simulink model "ISReferenceApplication"  (R2019b)
settings: Solver=VariableStepAuto  StartTime=0.0  StopTime=10.0  RelTol=1e-3
undefined symbols (not defined in the file or in its folder): C_Brake, C_Final, C_Front, C_Middle, C_out_Brake, C_out_Final, C_out_Front, C_out_Middle, Co, Cso, D_out_Brake, D_out_Final, D_out_Front, D_out_Middle, Downshift_Speeds, F, F_Brake, F_Final, F_Front, F_Middle, Fs, G_Brake, G_Final, G_Front, G_Middle, G_sys_Brake, G_sys_Final, G_sys_Front, G_sys_Middle, Gd, Gd_Brake, Gd_Final, Gsd, h, H_Brake, H_Final, H_Front, H_Middle, H_sys_Brake, H_sys_Final, H_sys_Front, H_sys_Middle, Hd, Hd_Brake, Hd_Final, Hsd, JE, JE_Brake, JE_Final, JE_Front, JE_Middle, JEs, JF_part, JF_part_Brake, JF_part_Final, JF_parts, Ld, Ld_Brake, Ld_Final, Ld_Front ... (+21)
libraries: simulink x5, autolibutils x3, sim3dlib x2, vehdynlibviscommon x1
(part 4 of 4)

== matlab function ISReferenceApplication/Final Observer2/Subsystem/Pose updete k/Update ==
  settings: updateMethod=DISCRETE  sampleTime=Ts
  data: Rs_V_now input; Rs_Y_now input; XYline input; XYplot input; XYplot_sim input; Last_XYplot_sim input; Velocity_sim input; Last_Velocity_sim input; Heading_sim input; Last_Heading_sim input; Tsim input; Last_Heading_end input; Velocity_updated output; Heading_updated output [1..5]; Heading_end output
function [Velocity_updated, Heading_updated, Heading_end] = Y_update(Rs_V_now, Rs_Y_now, ...
        XYline, XYplot, XYplot_sim, Last_XYplot_sim, Velocity_sim, Last_Velocity_sim, Heading_sim, Last_Heading_sim, ... 
    Tsim, Last_Heading_end)
    disp(sprintf('Simulation time : %2.1f sec',Tsim)) 
    Np = 5; Ts = 0.1;
    Heading_updated = zeros(Np,1); Velocity_updated = zeros(Np,1);Heading_end = 0;
    coder.extrinsic('intersections');
    coder.extrinsic('P2YV');
%     coder.varsize('Velocity_updated_tmp',[5 1]);
%     coder.varsize('Heading_updated_tmp',[5 1]);
     if Tsim == 0 
        plot(XYline(:,2),XYline(:,1),'black');
    end
   

%%Create half-circle    

    N = 30;
    theta = zeros(Np-1,N+1); Veh_circle = zeros(N+1,(Np-1)*2); 
    xp = zeros(1,N+1); yp = zeros(1,N+1); X = [];  Y = []; X_tmp = 0; Y_tmp = 0;
    lookahead = zeros(Np-1,1);
    
    XYplot_sim_tmp = XYplot_sim;    

%     if Velocity_sim > 0.5
        Velocity_ahead = [Velocity_sim; Rs_V_now(2:Np-1,:)];
%     else
%         Velocity_ahead = Rs_V_now;
%     end

    lookahead = Velocity_ahead*Ts;
    Headngahead = [Heading_sim; Rs_Y_now(2:Np-1,:)];
%     lookahead = [1; 1.5; 2; 2.5; 3];
        
    for j = 1:Np-1        
        theta = Headngahead(j,:)-pi/4 : pi/2/N : Headngahead(j,:)+pi/4;
        xp = lookahead(j,:)*cos(theta) + XYplot_sim_tmp(1,:)*ones(1,length(theta));
        yp = lookahead(j,:)*sin(theta) + XYplot_sim_tmp(2,:)*ones(1,length(theta));
        Veh_circle(:,2*j-1:2*j) = [xp' yp'];
       
    %Find the intersection    
         
        [X_tmp, Y_tmp] = intersections(XYplot(:,1), XYplot(:,2), Veh_circle(:,2*j-1), Veh_circle(:,2*j),0); 
        
        if X_tmp == 0 && Y_tmp == 0
%             X = X_tmp(1:j-1,:);
%             Y = Y_tmp(1:j-1,:);
            break;
        end

        X = [X; X_tmp];
        Y = [Y; Y_tmp];   
        XYplot_sim_tmp = [X_tmp; Y_tmp];
        
    end 
    
%%Obtain predict Velocity and Heading angle
   
  
    
    X = [Last_XYplot_sim(1,:); XYplot_sim(1,:); X];
    Y = [Last_XYplot_sim(2,:); XYplot_sim(2,:); Y];
    Vx0 = Last_Velocity_sim*cos(Last_Heading_sim);
    Vy0 = Last_Velocity_sim*sin(Last_Heading_sim);
    Yaw0 = Last_Heading_sim;
     
    T_sample = []; 
    for j = 1:length(X)
        T_sample = [T_sample; Tsim+(j-1)*Ts];
    end
    
   [Velocity_updated, Heading_updated] = P2YV(0, T_sample , X , Y , Vx0 , Vy0 , Yaw0, Np, Last_Heading_end );
   Heading_end = Heading_updated(end,:);

%     Heading_tmp_end = atan2(XYplot(end,2)-XYplot_sim(2,:), XYplot(end,1)-XYplot_sim(1,:));
% 
%     if  ((Heading_tmp_end - Heading_tmp_end_delay) < -5/3*pi) % Angle compensation
%         Heading_flag_end = Heading_flag_end + 1;
%     elseif ((Heading_tmp_end - Heading_tmp_end_delay) > 5/3*pi)
%         Heading_flag_end = Heading_flag_end - 1;
%     end
%     
%     if flag == 1
%         Heading_updated(1:end) = Heading_tmp_end + Heading_flag_end*2*pi;
%     end
%     if Tsim == 1.5
%         figure();
%         plot(XYplot(:,2),XYplot(:,1),'black-');
%         hold on;
%         plot(XYplot_sim(2,:),XYplot_sim(1,:),'b o');
%         plot(Veh_circle(:,2), Veh_circle(:,1),'b-');
%         plot(Veh_circle(:,4), Veh_circle(:,3),'b-');
%         plot(Veh_circle(:,6), Veh_circle(:,5),'b-');
%         plot(Veh_circle(:,8), Veh_circle(:,7),'b-');
%         plot(Veh_circle(:,10), Veh_circle(:,9),'b-');
%         plot(Y, X,'r x');
%     end

end

== matlab function ISReferenceApplication/Final Observer2/Subsystem/VH2P/YV2P ==
  data: Velocity input; Yaw input; LastVelocity input; LastYaw input; Tsim input; LastTsim input; Lastpostion input; Position output
function Position  = YV2P(Velocity, Yaw,  LastVelocity, LastYaw, Tsim, LastTsim, Lastpostion)
if Tsim >= 0.1
    Position = zeros(2,1);
    X0 = Lastpostion(1,:); Y0 = Lastpostion(2,:);
    Vx = [LastVelocity*cos(LastYaw); Velocity*cos(Yaw)];
    Vy = [LastVelocity*sin(LastYaw); Velocity*sin(Yaw)];
    Yaw_sim = [LastYaw; Yaw];
    T_sample =[LastTsim; Tsim];
    [ X_tmp, Y_tmp] = YV2P( T_sample, X0, Y0, Vx, Vy, Yaw_sim, zeros(2,1) );
    Position = [X_tmp(end,:); Y_tmp(end,:)];
else
    Position = [0; 0];
end

end

== matlab function ISReferenceApplication/Final Observer2/Subsystem/YV_update_Np/MATLAB Function2 ==
  data: XY_ref input; Velocity_updated output; XY_sim input; LastXY_sim input; Velocity_sim input; LastVelocity_sim input; Yaw_sim input; LastYaw_sim input; Tsim input; Heading_updated output
function [Velocity_updated, Heading_updated] = VY_update(XY_ref, XY_sim, LastXY_sim, Velocity_sim, LastVelocity_sim, Yaw_sim, LastYaw_sim, Tsim)
    disp(sprintf('Simulation time : %2.1f sec',Tsim)) 
 Ts = 0.1;
% Np = 6;
 Np = 6;

 Heading_updated = zeros(Np,1); Velocity_updated = zeros(Np,1);
coder.extrinsic('P2YV');
% T_sample = [Tsim-0.01; Tsim; Tsim+0.01];
% X = [LastXY_sim(1); XY_sim(1); XY_ref(1,:)];
% Y = [LastXY_sim(2); XY_sim(2); XY_ref(2,:)];

% T_sample = [Tsim-0.01; Tsim; Tsim+0.01; Tsim+0.02];
% X = [LastXY_sim(1); XY_sim(1); XY_ref(1,:); XY_ref(3,:)];
% Y = [LastXY_sim(2); XY_sim(2); XY_ref(2,:); XY_ref(4,:)];

T_sample = []; 
for j = 1:Np+1
    T_sample = [T_sample; Tsim+(j-1)*Ts];
end
X = [];
for i = 1:Np
    X = [X; XY_ref(2*i-1,:)];
end
Y = [];
for i = 1:Np
    Y = [Y; XY_ref(2*i,:)];
end

X = [XY_sim(1,:); X];
Y = [XY_sim(2,:); Y];   
Vx0 = Velocity_sim*cos(Yaw_sim);
Vy0 = Velocity_sim*sin(Yaw_sim);
Yaw0 = Yaw_sim;

[Velocity_updated, Heading_updated] = P2YV(0,0, T_sample , X , Y , Vx0 , Vy0 , Yaw0, Np, 0, 0 );

end

== matlab function ISReferenceApplication/Final Observer2/Subsystem/VH2P/MATLAB Function1 ==
  data: select_model input; tri output
function tri = trigger(select_model)
tri = 0;
if  select_model ==3
    tri=1;
else
    tri=0;
end
end

== matlab function ISReferenceApplication/Middle Observer3/MATLAB Function ==
  data: select_model input; tri output
function tri = trigger(select_model)
tri = 0;
if select_model==2 
    tri=1;
else
    tri=0;
end
end

== matlab function ISReferenceApplication/Middle Observer3/Subsystem/MATLAB Function ==
  data: select_model input; tri output
function tri = trigger(select_model)
tri = 0;
if select_model == 2 
    tri=1;
else
    tri=0;
end
end

== matlab function ISReferenceApplication/Middle Observer3/Subsystem/VH2P/MATLAB Function ==
  data: select_model input; tri output
function tri = trigger(select_model)
tri = 0;
if select_model == 2 
    tri=1;
else
    tri=0;
end
end

== matlab function ISReferenceApplication/Middle Observer2/Subsystem/MATLAB Function1 ==
  data: select_model input; tri output
function tri = trigger(select_model)
tri = 0;
if select_model == 1
    tri=1;
else
    tri=0;
end
end

== matlab function ISReferenceApplication/Middle Observer2/Subsystem/VH2P/MATLAB Function1 ==
  data: select_model input; tri output
function tri = trigger(select_model)
tri = 0;
if select_model == 1
    tri=1;
else
    tri=0;
end
end

== matlab function ISReferenceApplication/Final Observer1/MATLAB Function1 ==
  data: select_model input; tri output
function tri = trigger(select_model)
tri = 0;
if select_model == 4%% || select_model ==3
    tri=1;
else
    tri=0;
end
end

== matlab function ISReferenceApplication/Final Observer1/Subsystem/MATLAB Function1 ==
  data: select_model input; tri output
function tri = trigger(select_model)
tri = 0;
if  select_model ==4
    tri=1;
else
    tri=0;
end
end

== matlab function ISReferenceApplication/Final Observer1/Subsystem/Mpc_Simulator_Final/MATLAB Function ==
  data: Ref output; JE input; U output; M input; Np input; phi input; Qc input; Fxh input; Yup input; Vup input; Rs input; Tsim input; Upd_end input; u input
function [Ref,U] = HQP(JE,M,Np,phi,Qc,Fxh,Yup,Vup,Rs,Tsim,Upd_end,u)

% if Tsim < 6.27 %(sec)
%     u1_max =  5/3*pi; u1_min = -5/3*pi;
%     u2_max =  0.3; u2_min = -1;
%     du1_inc =  1*5/3*pi; 
%     du1_dec =  1*5/3*pi; 
%     du2_inc =  0.03;
%     du2_dec =  0.03;
% else 
    u1_max =  5/3*pi; u1_min = -5/3*pi;
    u2_max =  1; u2_min = -1;
    du1_inc =  1*5/3*pi;
    du1_dec =  1*5/3*pi;
    du2_inc =  1;
    du2_dec =  1;
% end
% du1_max =  0.1*abs(Fxh(1,:)); 
% du2_max =  0.05*abs(Fxh(1,:)); 
% Y1_min = Rs(1,:) - 2;%V
% Y1_max = Rs(1,:) + 2;%V
% Y2_min = Rs(2,:) - 0.2;%Y
% Y2_max = Rs(2,:) + 0.2;%Y
% 
% Y1_min = -10;%V
% Y2_min = -100;%Y
% Y1_max = 50;%V
% Y2_max = 100;%Y

% Y_max = [];
% Y_min = [];
% for i = 1:Np
%     Y_max = [Y_max;[Y1_max;Y2_max]];
%     Y_min = [Y_min;[Y1_min;Y2_min]];
% end

U_max = []; U_min = [];
for i = 1:Np
    U_max = [U_max; [u1_max; u2_max]];
    U_min = [U_min; [-u1_min; -u2_min]];
end

dU_plus = []; dU_minus = [];
for i = 1:Np
    dU_plus = [dU_plus; [u(1) + du1_inc; u(2) + du2_inc]];
    dU_minus = [dU_minus; [-u(1) + du1_dec; -u(2) + du2_dec;]];
end
rr = [U_max;
      U_min;
      dU_plus;
      dU_minus;          
     ];
 
% rr_y = [Y_max - Fxh;
%        -Y_min + Fxh;
%        ];
N = [];
N = rr; 
% N = [rr;rr_y];


if Tsim > 0 && Tsim < Upd_end
%     for i = 1: Np
%         Rs(2*i,:) = Yup(i,:);
%         Rs(2*i-1,:) = Vup(i,:);
%     end
% elseif Tsim >= 65
%     for i = 1: Np
%         Rs(2*i,:) = Yup(i,:);
% %         Rs(2*i-1,:) = Vup(i,:);
%     end
end


JF = -2*phi'*Qc*(Rs-Fxh);
[uc,lambda]= HQP(JE,JF,M,N);
U = uc(1:2);
% if Tsim <= Timetochange
%     U(1,:) = 1e-9;
% end
Ref = Rs(1:2,:);
% lambda
end

== matlab function ISReferenceApplication/Final Observer1/Subsystem/Pose updete k/Update ==
  settings: updateMethod=DISCRETE  sampleTime=Ts
  data: Rs_V_now input; Rs_Y_now input; XYline input; XYplot input; XYplot_sim input; Last_XYplot_sim input; Velocity_sim input; Last_Velocity_sim input; Heading_sim input; Last_Heading_sim input; Tsim input; Last_Heading_end input; Velocity_updated output; Heading_updated output [1..5]; Heading_end output
function [Velocity_updated, Heading_updated, Heading_end] = Y_update(Rs_V_now, Rs_Y_now, ...
        XYline, XYplot, XYplot_sim, Last_XYplot_sim, Velocity_sim, Last_Velocity_sim, Heading_sim, Last_Heading_sim, ... 
    Tsim, Last_Heading_end)
    disp(sprintf('Simulation time : %2.1f sec',Tsim)) 
    Np = 5; Ts = 0.1;
    Heading_updated = zeros(Np,1); Velocity_updated = zeros(Np,1);Heading_end = 0;
    coder.extrinsic('intersections');
    coder.extrinsic('P2YV');
%     coder.varsize('Velocity_updated_tmp',[5 1]);
%     coder.varsize('Heading_updated_tmp',[5 1]);
     if Tsim == 0 
        plot(XYline(:,2),XYline(:,1),'black');
    end
   

%%Create half-circle    

    N = 30;
    theta = zeros(Np-1,N+1); Veh_circle = zeros(N+1,(Np-1)*2); 
    xp = zeros(1,N+1); yp = zeros(1,N+1); X = [];  Y = []; X_tmp = 0; Y_tmp = 0;
    lookahead = zeros(Np-1,1);
    
    XYplot_sim_tmp = XYplot_sim;    

%     if Velocity_sim > 0.5
        Velocity_ahead = [Velocity_sim; Rs_V_now(2:Np-1,:)];
%     else
%         Velocity_ahead = Rs_V_now;
%     end

    lookahead = Velocity_ahead*Ts;
    Headngahead = [Heading_sim; Rs_Y_now(2:Np-1,:)];
%     lookahead = [1; 1.5; 2; 2.5; 3];
        
    for j = 1:Np-1        
        theta = Headngahead(j,:)-pi/4 : pi/2/N : Headngahead(j,:)+pi/4;
        xp = lookahead(j,:)*cos(theta) + XYplot_sim_tmp(1,:)*ones(1,length(theta));
        yp = lookahead(j,:)*sin(theta) + XYplot_sim_tmp(2,:)*ones(1,length(theta));
        Veh_circle(:,2*j-1:2*j) = [xp' yp'];
       
    %Find the intersection    
         
        [X_tmp, Y_tmp] = intersections(XYplot(:,1), XYplot(:,2), Veh_circle(:,2*j-1), Veh_circle(:,2*j),0); 
        
        if X_tmp == 0 && Y_tmp == 0
%             X = X_tmp(1:j-1,:);
%             Y = Y_tmp(1:j-1,:);
            break;
        end

        X = [X; X_tmp];
        Y = [Y; Y_tmp];   
        XYplot_sim_tmp = [X_tmp; Y_tmp];
        
    end 
    
%%Obtain predict Velocity and Heading angle
   
  
    
    X = [Last_XYplot_sim(1,:); XYplot_sim(1,:); X];
    Y = [Last_XYplot_sim(2,:); XYplot_sim(2,:); Y];
    Vx0 = Last_Velocity_sim*cos(Last_Heading_sim);
    Vy0 = Last_Velocity_sim*sin(Last_Heading_sim);
    Yaw0 = Last_Heading_sim;
     
    T_sample = []; 
    for j = 1:length(X)
        T_sample = [T_sample; Tsim+(j-1)*Ts];
    end
    
   [Velocity_updated, Heading_updated] = P2YV(0, T_sample , X , Y , Vx0 , Vy0 , Yaw0, Np, Last_Heading_end );
   Heading_end = Heading_updated(end,:);

%     Heading_tmp_end = atan2(XYplot(end,2)-XYplot_sim(2,:), XYplot(end,1)-XYplot_sim(1,:));
% 
%     if  ((Heading_tmp_end - Heading_tmp_end_delay) < -5/3*pi) % Angle compensation
%         Heading_flag_end = Heading_flag_end + 1;
%     elseif ((Heading_tmp_end - Heading_tmp_end_delay) > 5/3*pi)
%         Heading_flag_end = Heading_flag_end - 1;
%     end
%     
%     if flag == 1
%         Heading_updated(1:end) = Heading_tmp_end + Heading_flag_end*2*pi;
%     end
%     if Tsim == 1.5
%         figure();
%         plot(XYplot(:,2),XYplot(:,1),'black-');
%         hold on;
%         plot(XYplot_sim(2,:),XYplot_sim(1,:),'b o');
%         plot(Veh_circle(:,2), Veh_circle(:,1),'b-');
%         plot(Veh_circle(:,4), Veh_circle(:,3),'b-');
%         plot(Veh_circle(:,6), Veh_circle(:,5),'b-');
%         plot(Veh_circle(:,8), Veh_circle(:,7),'b-');
%         plot(Veh_circle(:,10), Veh_circle(:,9),'b-');
%         plot(Y, X,'r x');
%     end

end

== matlab function ISReferenceApplication/Final Observer1/Subsystem/VH2P/MATLAB Function1 ==
  data: select_model input; tri output
function tri = trigger(select_model)
tri = 0;
if  select_model ==4
    tri=1;
else
    tri=0;
end
end

== matlab function ISReferenceApplication/Final Observer1/Subsystem/VH2P/YV2P ==
  data: Velocity input; Yaw input; LastVelocity input; LastYaw input; Tsim input; LastTsim input; Lastpostion input; Position output
function Position  = YV2P(Velocity, Yaw,  LastVelocity, LastYaw, Tsim, LastTsim, Lastpostion)
if Tsim >= 0.1
    Position = zeros(2,1);
    X0 = Lastpostion(1,:); Y0 = Lastpostion(2,:);
    Vx = [LastVelocity*cos(LastYaw); Velocity*cos(Yaw)];
    Vy = [LastVelocity*sin(LastYaw); Velocity*sin(Yaw)];
    Yaw_sim = [LastYaw; Yaw];
    T_sample =[LastTsim; Tsim];
    [ X_tmp, Y_tmp] = YV2P( T_sample, X0, Y0, Vx, Vy, Yaw_sim, zeros(2,1) );
    Position = [X_tmp(end,:); Y_tmp(end,:)];
else
    Position = [0; 0];
end

end

== matlab function ISReferenceApplication/Final Observer1/Subsystem/YV_update_Np/MATLAB Function2 ==
  data: XY_ref input; Velocity_updated output; XY_sim input; LastXY_sim input; Velocity_sim input; LastVelocity_sim input; Yaw_sim input; LastYaw_sim input; Tsim input; Heading_updated output
function [Velocity_updated, Heading_updated] = VY_update(XY_ref, XY_sim, LastXY_sim, Velocity_sim, LastVelocity_sim, Yaw_sim, LastYaw_sim, Tsim)
    disp(sprintf('Simulation time : %2.1f sec',Tsim)) 
 Ts = 0.1;
% Np = 6;
 Np = 6;

 Heading_updated = zeros(Np,1); Velocity_updated = zeros(Np,1);
coder.extrinsic('P2YV');
% T_sample = [Tsim-0.01; Tsim; Tsim+0.01];
% X = [LastXY_sim(1); XY_sim(1); XY_ref(1,:)];
% Y = [LastXY_sim(2); XY_sim(2); XY_ref(2,:)];

% T_sample = [Tsim-0.01; Tsim; Tsim+0.01; Tsim+0.02];
% X = [LastXY_sim(1); XY_sim(1); XY_ref(1,:); XY_ref(3,:)];
% Y = [LastXY_sim(2); XY_sim(2); XY_ref(2,:); XY_ref(4,:)];

T_sample = []; 
for j = 1:Np+1
    T_sample = [T_sample; Tsim+(j-1)*Ts];
end
X = [];
for i = 1:Np
    X = [X; XY_ref(2*i-1,:)];
end
Y = [];
for i = 1:Np
    Y = [Y; XY_ref(2*i,:)];
end

X = [XY_sim(1,:); X];
Y = [XY_sim(2,:); Y];   
Vx0 = Velocity_sim*cos(Yaw_sim);
Vy0 = Velocity_sim*sin(Yaw_sim);
Yaw0 = Yaw_sim;

[Velocity_updated, Heading_updated] = P2YV(0,0, T_sample , X , Y , Vx0 , Vy0 , Yaw0, Np, 0, 0 );

end
